simulink model "modnl_sim_template"  (R2015a)
settings: Solver=ode1  SolverMode=SingleTasking  StartTime=0.0  StopTime=10  FixedStep=0.01  RelTol=1e-3
values from neighbouring files (symbols this model uses):
  K = Zinf/(n^2*deltaVm)    (= 59.85)    [Exp4.m]
  Kp = 1.455    [Exp4.m]
  Kt = 0.0169    [Exp4.m]
  phi = K*n^2*Vm1 - wp1    (= 1.2)    [Exp4.m]
  T = 0.28    [Exp4.m]
settings Model: CovExternalEMLEnable=on  Creator=rpm  LastModifiedBy=rpm
settings DataIOCC: LimitDataPoints=off  SignalLoggingSaveFormat=ModelDataLogs  SaveOutput=off  SignalLogging=off  DSMLogging=off  SaveTime=off  TimeSaveName=t
settings OptimizationCC: ExpressionDepthLimit=2147483647  InitFltsAndDblsToZero=on
settings DebuggingCC: UnderspecifiedInitializationDetection=Classic  MergeDetectMultiDrivingBlocksExec=none  FcnCallInpInsideContextMsg=EnableAllAsWarning  StateNameClashWarn=warning
settings GRTTargetCC: CombineOutputUpdateFcns=off  GRTInterface=on

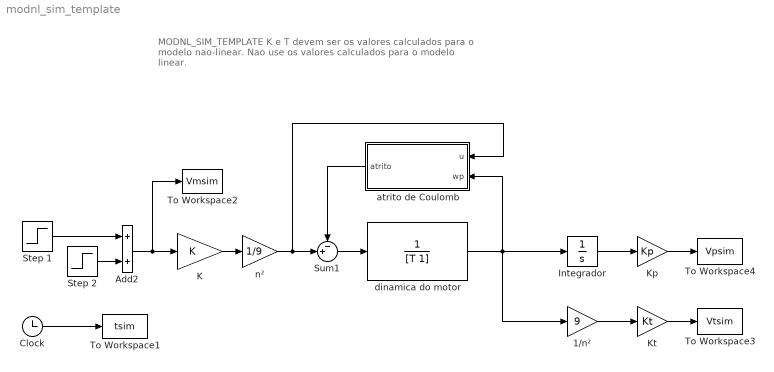
== system modnl_sim_template ==
  note: MODNL_SIM_TEMPLATE
      |
      | K e T devem ser os valores calculados para o
      | modelo nao-linear. Nao use os valores
      | calculados para o modelo linear.
  1/n² : Gain  Gain=9
  Add2 : Sum
  Clock : Clock
  Integrador : Integrator
  K : Gain  Gain=K
  Kp : Gain  Gain=Kp
  Kt : Gain  Gain=Kt
  Step 1 : Step  After=2  SampleTime=0
  Step 2 : Step  Time=5  After=2  SampleTime=0
  Sum1 : Sum  Inputs=-+|
  To Workspace1 : ToWorkspace  VariableName=tsim  SampleTime=-1
  To Workspace2 : ToWorkspace  VariableName=Vmsim  SampleTime=-1
  To Workspace3 : ToWorkspace  VariableName=Vtsim  SampleTime=-1
  To Workspace4 : ToWorkspace  VariableName=Vpsim  SampleTime=-1
  atrito de Coulomb : Subsystem  mask{phi=phi}
      mask Display: fprintf('phi = %3.1f', phi)
  dinamica do motor : TransferFcn  Denominator=[T 1]
  n² : Gain  Gain=1/9
  wires:
  dinamica do motor/1 -> 1/n²/1, Integrador/1, atrito de Coulomb/2(wp)
  Integrador/1 -> Kp/1
  Kt/1 -> To Workspace3/1
  Kp/1 -> To Workspace4/1
  K/1 -> n²/1
  n²/1 -> atrito de Coulomb/1(u), Sum1/2
  atrito de Coulomb/1(atrito) -> Sum1/1
  Sum1/1 -> dinamica do motor/1
  1/n²/1 -> Kt/1
  Add2/1 -> To Workspace2/1, K/1
  Step 1/1 -> Add2/1
  Step 2/1 -> Add2/2
  Clock/1 -> To Workspace1/1

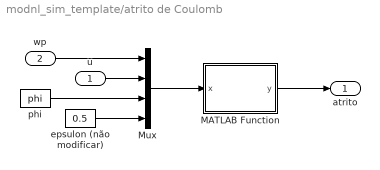
== system modnl_sim_template/atrito de Coulomb ==
  u : Inport
  wp : Inport  Port=2
  MATLAB Function : MATLAB Function  TreatAsAtomicUnit=on
      settings: PermitHierarchicalResolution=ParametersOnly
  Mux : Mux
  epsulon (não modificar) : Constant  Value=0.5
  phi : Constant  Value=phi
  atrito : Outport
  wires:
  u/1 -> Mux/2
  phi/1 -> Mux/3
  MATLAB Function/1(y) -> atrito/1
  wp/1 -> Mux/1
  epsulon (não modificar)/1 -> Mux/4
  Mux/1 -> MATLAB Function/1(x)

== matlab function modnl_sim_template/atrito de Coulomb/MATLAB Function ==
  data: x input size=4; y output size=1
function y = nl_coulomb(x)
% Atrito de Coulomb
% Para uso de nl_template.mdl

wp  = x(1); 
u   = x(2); 
phi = x(3); 
epsulon = x(4);

y = 0;

if wp > epsulon
    y = phi;
elseif wp < -epsulon
    y = -phi;
elseif wp >= 0
    y = min(phi,abs(u));
elseif wp < 0
    y = max(-phi,-abs(u));
end
